simulink model "EV3robot_model"  (R2017a)
settings: Solver=VariableStepAuto  StartTime=0.0  StopTime=40  RelTol=1e-3  EnableMultiTasking=on
values from neighbouring files (symbols this model uses):
  Km = 9.812    [Matrix_dictionary.m]
  Tm = 0.055    [Matrix_dictionary.m]
undefined symbols (not defined in the file or in its folder): COLden, COLnum, DiscIntNeverNeededParam, Steering_PID_D, Steering_PID_I, Steering_PID_P, Ts, Vm
libraries: simulink x6
settings Model: ExtModeTrigDuration=2  Creator=mwcant  LastModifiedBy=linany
settings SolverCC: PositivePriorityOrder=on
settings OptimizationCC: MaxStackSize=64
settings DebuggingCC: ParameterTunabilityLossMsg=error
settings HardwareCC: ProdBitPerPointer=32  ProdBitPerSizeT=32  ProdBitPerPtrDiffT=32  ProdLargestAtomicInteger=Long  ProdWordSize=32  ProdHWDeviceType=ARM Compatible->ARM 9
settings SFSimCC: MATLABDynamicMemAlloc=off
settings RTWCC: SystemTargetFile=ert.tlc  HardwareBoard=LEGO MINDSTORMS EV3  TLCOptions="-aInlineSetEventsForThisBaseRateFcn=TLC_FALSE -aSuppressMultiTaskScheduler=TLC_FALSE  -aRateBasedStepFcn=0"  TemplateMakefile=ert_default_tmf  Description=Embedded Coder  GenerateReport=on  Toolchain=Sourcery G++ Lite v2009q3  IncludeHyperlinkInReport=on  LaunchReport=on  GenerateTraceInfo=on  GenerateTraceReport=on  GenerateTraceReportSl=on  GenerateTraceReportSf=on  GenerateTraceReportEml=on
settings CodeAppCC: ForceParamTrailComments=on  IgnoreCustomStorageClasses=off  OperatorAnnotations=on  SimulinkDataObjDesc=on  SFDataObjDesc=on  MATLABFcnDesc=on  InsertBlockDesc=on  MATLABSourceComments=on
settings ERTTargetCC: MultiwordLength=2048  SupportContinuousTime=on  SupportVariableSizeSignals=on  ExtMode=on  ExtModeMexArgs='192.168.1.19' 0 17725

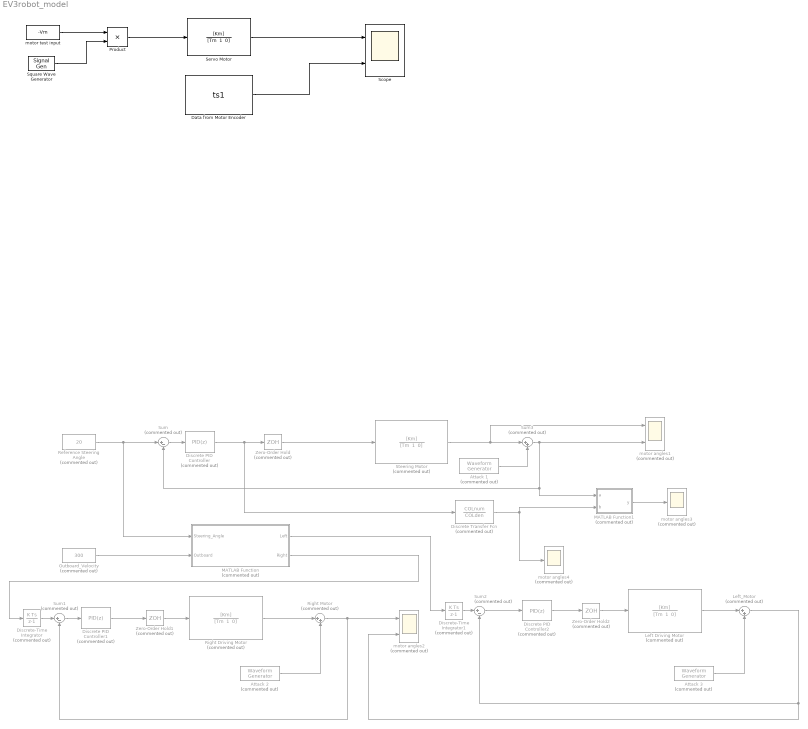
== system EV3robot_model ==
  Attack 1 : simulink/Sources/Waveform Generator  Commented=on  OutMin=[]  OutMax=[]  OutDataTypeStr=double  SelectedSignal=1  Signals=step('StepTime',5,'InitialValue',0,'FinalValue',5)#step('StepTime',10,'InitialValue',0,'FinalValue',-5)  BlockNames=MultiportSwitch_20c5d9b88be2448#MultiportSwitch_2ef32689821f40e  SampleTime=-1
      settings: SourceProductName=Simulink
  Attack 2 : simulink/Sources/Waveform Generator  Commented=on  OutMin=[]  OutMax=[]  OutDataTypeStr=double  SelectedSignal=1  Signals=step('StepTime',10,'InitialValue',0,'FinalValue',500)  BlockNames=MultiportSwitch_f8fa683eb519425  SampleTime=-1
      settings: SourceProductName=Simulink
  Attack 3 : simulink/Sources/Waveform Generator  Commented=on  OutMin=[]  OutMax=[]  OutDataTypeStr=double  SelectedSignal=1  BlockNames=MultiportSwitch_e3df3653d217406  SampleTime=0.1
      settings: SourceProductName=Simulink
  "Data from Motor Encoder " : FromWorkspace  VariableName=ts1  SampleTime=0
      mask Display: image('Picture1.jpg');
  Discrete Transfer Fcn : DiscreteTransferFcn  Commented=on  Numerator=COLnum  Denominator=COLden  SampleTime=Ts
  Discrete PID Controller : simulink/Continuous/PID Controller  Commented=on  Controller=PID  TimeDomain=Discrete-time  SampleTime=Ts  IntegratorMethod=Forward Euler  FilterMethod=Forward Euler  Form=Parallel  UseFilter=off  ControllerParametersSource=internal  P=Steering_PID_P  I=Steering_PID_I  D=Steering_PID_D  N=100  InitialConditionSource=internal  InitialConditionForIntegrator=0  InitialConditionForFilter=0  ExternalReset=none  LimitOutput=off  UpperSaturationLimit=inf  LowerSaturationLimit=-inf  LinearizeAsGain=off  AntiWindupMode=none  Kb=1  TrackingMode=off  Kt=1  PParamMin=[]  PParamMax=[]  IParamMin=[]  IParamMax=[]  DParamMin=[]  DParamMax=[]  NParamMin=[]  NParamMax=[]  KbParamMin=[]  KbParamMax=[]  KtParamMin=[]  KtParamMax=[]  POutMin=[]  POutMax=[]  IOutMin=[]  IOutMax=[]  DOutMin=[]  DOutMax=[]  NOutMin=[]  NOutMax=[]  KbOutMin=[]  KbOutMax=[]  KtOutMin=[]  KtOutMax=[]  IntegratorOutMin=[]  IntegratorOutMax=[]  FilterOutMin=[]  FilterOutMax=[]  SumOutMin=[]  SumOutMax=[]  SumI1OutMin=[]  SumI1OutMax=[]  SumI2OutMin=[]  SumI2OutMax=[]  SumI3OutMin=[]  SumI3OutMax=[]  SumDOutMin=[]  SumDOutMax=[]  SaturationOutMin=[]  SaturationOutMax=[]  IntegratorContinuousStateAttributes=''  IntegratorStateMustResolveToSignalObject=off  IntegratorRTWStateStorageClass=Auto  FilterContinuousStateAttributes=''  FilterStateMustResolveToSignalObject=off  FilterRTWStateStorageClass=Auto  DifferentiatorICPrevScaledInput=0  DifferentiatorOutMin=[]  DifferentiatorOutMax=[]  InitialConditionSetting=State (most efficient)
  Discrete PID Controller1 : simulink/Continuous/PID Controller  Commented=on  Controller=PID  TimeDomain=Discrete-time  SampleTime=Ts  IntegratorMethod=Forward Euler  FilterMethod=Forward Euler  Form=Parallel  UseFilter=off  ControllerParametersSource=internal  P=0.25  I=0  D=0  N=100  InitialConditionSource=internal  InitialConditionForIntegrator=0  InitialConditionForFilter=0  ExternalReset=none  LimitOutput=off  UpperSaturationLimit=inf  LowerSaturationLimit=-inf  LinearizeAsGain=off  AntiWindupMode=none  Kb=1  TrackingMode=off  Kt=1  PParamMin=[]  PParamMax=[]  IParamMin=[]  IParamMax=[]  DParamMin=[]  DParamMax=[]  NParamMin=[]  NParamMax=[]  KbParamMin=[]  KbParamMax=[]  KtParamMin=[]  KtParamMax=[]  POutMin=[]  POutMax=[]  IOutMin=[]  IOutMax=[]  DOutMin=[]  DOutMax=[]  NOutMin=[]  NOutMax=[]  KbOutMin=[]  KbOutMax=[]  KtOutMin=[]  KtOutMax=[]  IntegratorOutMin=[]  IntegratorOutMax=[]  FilterOutMin=[]  FilterOutMax=[]  SumOutMin=[]  SumOutMax=[]  SumI1OutMin=[]  SumI1OutMax=[]  SumI2OutMin=[]  SumI2OutMax=[]  SumI3OutMin=[]  SumI3OutMax=[]  SumDOutMin=[]  SumDOutMax=[]  SaturationOutMin=[]  SaturationOutMax=[]  IntegratorContinuousStateAttributes=''  IntegratorStateMustResolveToSignalObject=off  IntegratorRTWStateStorageClass=Auto  FilterContinuousStateAttributes=''  FilterStateMustResolveToSignalObject=off  FilterRTWStateStorageClass=Auto  DifferentiatorICPrevScaledInput=0  DifferentiatorOutMin=[]  DifferentiatorOutMax=[]  InitialConditionSetting=State (most efficient)
  Discrete PID Controller2 : simulink/Continuous/PID Controller  Commented=on  Controller=PID  TimeDomain=Discrete-time  SampleTime=Ts  IntegratorMethod=Forward Euler  FilterMethod=Forward Euler  Form=Parallel  UseFilter=off  ControllerParametersSource=internal  P=0.25  I=0  D=0  N=100  InitialConditionSource=internal  InitialConditionForIntegrator=0  InitialConditionForFilter=0  ExternalReset=none  LimitOutput=off  UpperSaturationLimit=inf  LowerSaturationLimit=-inf  LinearizeAsGain=off  AntiWindupMode=none  Kb=1  TrackingMode=off  Kt=1  PParamMin=[]  PParamMax=[]  IParamMin=[]  IParamMax=[]  DParamMin=[]  DParamMax=[]  NParamMin=[]  NParamMax=[]  KbParamMin=[]  KbParamMax=[]  KtParamMin=[]  KtParamMax=[]  POutMin=[]  POutMax=[]  IOutMin=[]  IOutMax=[]  DOutMin=[]  DOutMax=[]  NOutMin=[]  NOutMax=[]  KbOutMin=[]  KbOutMax=[]  KtOutMin=[]  KtOutMax=[]  IntegratorOutMin=[]  IntegratorOutMax=[]  FilterOutMin=[]  FilterOutMax=[]  SumOutMin=[]  SumOutMax=[]  SumI1OutMin=[]  SumI1OutMax=[]  SumI2OutMin=[]  SumI2OutMax=[]  SumI3OutMin=[]  SumI3OutMax=[]  SumDOutMin=[]  SumDOutMax=[]  SaturationOutMin=[]  SaturationOutMax=[]  IntegratorContinuousStateAttributes=''  IntegratorStateMustResolveToSignalObject=off  IntegratorRTWStateStorageClass=Auto  FilterContinuousStateAttributes=''  FilterStateMustResolveToSignalObject=off  FilterRTWStateStorageClass=Auto  DifferentiatorICPrevScaledInput=0  DifferentiatorOutMin=[]  DifferentiatorOutMax=[]  InitialConditionSetting=State (most efficient)
  Discrete-Time Integrator : DiscreteIntegrator  Commented=on  InitialConditionSetting=State (most efficient)  SampleTime=-1  ICPrevOutput=DiscIntNeverNeededParam  ICPrevScaledInput=DiscIntNeverNeededParam
  Discrete-Time Integrator1 : DiscreteIntegrator  Commented=on  InitialConditionSetting=State (most efficient)  SampleTime=-1  ICPrevOutput=DiscIntNeverNeededParam  ICPrevScaledInput=DiscIntNeverNeededParam
  Left Driving Motor : TransferFcn  Commented=on  Numerator=[Km]  Denominator="[Tm  1  0]"
      mask Display: image('Picture1.jpg');
  Left_Motor : Sum  Commented=on  Inputs=|++
  MATLAB Function : MATLAB Function  Commented=on  TreatAsAtomicUnit=on
  MATLAB Function1 : MATLAB Function  Commented=on  TreatAsAtomicUnit=on
  Outboard_Velocity : Constant  Commented=on  Value=300
  Product : Product
  Reference Steering Angle : Constant  Commented=on  Value=20
  Right Driving Motor : TransferFcn  Commented=on  Numerator=[Km]  Denominator="[Tm  1  0]"
      mask Display: image('Picture1.jpg');
  Right Motor : Sum  Commented=on  Inputs=|++
  Scope : Scope  NumInputPorts=2
  Servo Motor : TransferFcn  Numerator=[Km]  Denominator="[Tm  1  0]"
  Square Wave Generator : SignalGenerator  WaveForm=square  Frequency=1/40
  Steering Motor : TransferFcn  Commented=on  Numerator=[Km]  Denominator="[Tm  1  0]"
      mask Display: image('Picture1.jpg');
  Sum : Sum  Commented=on  Inputs=|+-
  Sum1 : Sum  Commented=on  Inputs=|+-
  Sum2 : Sum  Commented=on  Inputs=|+-
  Sum3 : Sum  Commented=on  Inputs=|++
  Zero-Order Hold : ZeroOrderHold  Commented=on  SampleTime=-1
  Zero-Order Hold1 : ZeroOrderHold  Commented=on  SampleTime=-1
  Zero-Order Hold2 : ZeroOrderHold  Commented=on  SampleTime=-1
  motor angles1 : Scope  Commented=on  NumInputPorts=2
  motor angles2 : Scope  Commented=on  NumInputPorts=2
  motor angles3 : Scope  Commented=on
  motor angles4 : Scope  Commented=on
  motor test input : Constant  Value=-Vm
  wires:
  Discrete PID Controller/1 -> Discrete Transfer Fcn/1, Zero-Order Hold/1
  Reference Steering Angle/1 -> Sum/1, MATLAB Function/1(Steering_Angle)
  Sum/1 -> Discrete PID Controller/1
  MATLAB Function/2(Right) -> Discrete-Time Integrator/1
  MATLAB Function/1(Left) -> Discrete-Time Integrator1/1
  Sum1/1 -> Discrete PID Controller1/1
  Discrete PID Controller1/1 -> Zero-Order Hold1/1
  Sum2/1 -> Discrete PID Controller2/1
  Discrete PID Controller2/1 -> Zero-Order Hold2/1
  Zero-Order Hold2/1 -> Left Driving Motor/1
  Zero-Order Hold1/1 -> Right Driving Motor/1
  Right Motor/1 -> motor angles2/1, Sum1/2
  Left_Motor/1 -> Sum2/2, motor angles2/2
  Steering Motor/1 -> motor angles1/1, Sum3/1
  Sum3/1 -> MATLAB Function1/1(a), Sum/2, motor angles1/2
  Right Driving Motor/1 -> Right Motor/1
  Attack 2/1 -> Right Motor/2
  Left Driving Motor/1 -> Left_Motor/1
  Attack 3/1 -> Left_Motor/2
  Attack 1/1 -> Sum3/2
  Outboard_Velocity/1 -> MATLAB Function/2(Outboard)
  Discrete-Time Integrator/1 -> Sum1/1
  Discrete-Time Integrator1/1 -> Sum2/1
  Discrete Transfer Fcn/1 -> motor angles4/1, MATLAB Function1/2(b)
  Zero-Order Hold/1 -> Steering Motor/1
  MATLAB Function1/1(y) -> motor angles3/1
  Product/1 -> Servo Motor/1
  motor test input/1 -> Product/1
  Square Wave Generator/1 -> Product/2
  Servo Motor/1 -> Scope/1
  "Data from Motor Encoder "/1 -> Scope/2

== matlab function EV3robot_model/MATLAB Function1 ==
  data: a input; y output; b input
function y = fcn(a ,b)

if abs(a-b) >= 4
    y = 1;
else
    y = 0;
end
end

== matlab function EV3robot_model/MATLAB Function ==
  data: Steering_Angle input; Left output; Outboard input; Right output
function [Left,Right]= Inner_Velocity_Calculator(Steering_Angle, Outboard)
Inner_Speed = NXT_Demo_Speed_ratio (Steering_Angle, Outboard);
if Steering_Angle >= 0
    Right = Outboard;
    Left = Inner_Speed;
else 
    Right = Inner_Speed;
    Left = Outboard;
end
